simulink model "DC_Motor"  (R2021a)
settings: Solver=FixedStepAuto  StartTime=0.0  StopTime=10.0  FixedStep=25e-6  RelTol=1e-3
undefined symbols (not defined in the file): B, kephi, kphi, Ra, tau_a, tau_m, TL, Va
libraries: simulink_extras x2, spspowerguiLib x1
settings Model: Creator=lesinko morris  LastModifiedBy=lesinko morris
settings DataIOCC: SaveOutput=off  SignalLogging=off  SaveTime=off  ReturnWorkspaceOutputs=off  LoggingToFile=on

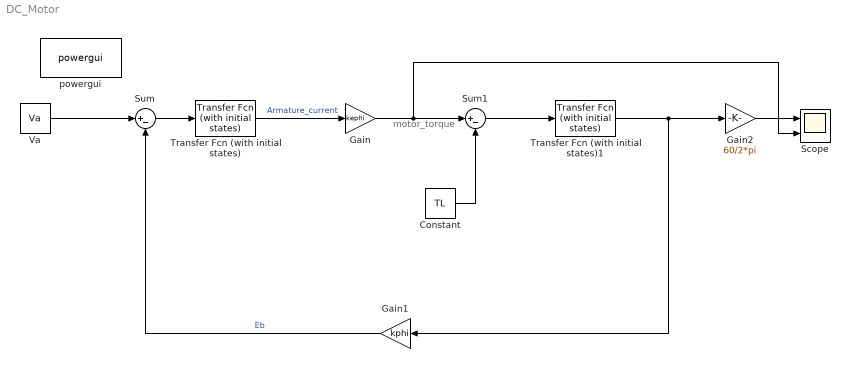
== system DC_Motor ==
  note: motor_torque
  Constant : Constant  Value=TL
  Gain : Gain  Gain=kephi
  Gain1 : Gain  Gain=kphi
  Gain2 : Gain  Gain=60/2*pi
  Scope : Scope  NumInputPorts=2
  Sum : Sum  Inputs=|+-
  Sum1 : Sum  Inputs=|+-
  Transfer Fcn (with initial states) : simulink_extras/Additional Linear/Transfer Fcn (with initial states)  N=[1/Ra]  D=[tau_a 1]  X0=.5
  Transfer Fcn (with initial states)1 : simulink_extras/Additional Linear/Transfer Fcn (with initial states)  N=[1/B]  D=[tau_m 1]  X0=.5
  Va : Constant  Value=Va
  powergui : spspowerguiLib/powergui  Priority=1  SimulationMode=Continuous  SampleTime=50e-6  frequency=60  Iterations=50  frequencyindice=60  Pbase=100e6  ErrMax=1e-4  UnitsV=kV  UnitsW=MW  buscounter=0  FunctionMessages=off  echomessages=off  EnableUseOfTLC=off  CurrentSourceSwitches=off  DisableSnubberDevices=off  DisableRonSwitches=off  DisableVfSwitches=off  DisplayEquations=off  AutomaticDiscreteSolvers=off  SolverType=Tustin/Backward Euler (TBE)  Interpol=off  ExternalGateDelay=off  methode=off  Ts=100  x0status=blocks  SPID=on  SwTol=0  HookPort=off  NonlinearTolerance=1e-4  nMaxIteration=100  ContinueOnMaxIteration=off  RestoreLinks=warning  ResistiveCurrentMeasurement=off  Frange=[0:2:500]  Ylog=off  Xlog=on  ShowGrid=off  save=off  variable=ZData  structure=0  ZoomFFT=off  StartTime=0.0  cycles=1  DisplayStyle=1  fundamental=60  FreqAxis=off  MaxFrequency=1000  frequencyindicesteady=1  RmsSteady=1  display=off
  wires:
  Va/1 -> Sum/1
  Sum/1 -> Transfer Fcn (with initial states)/1
  Transfer Fcn (with initial states)/1 -> Gain/1  "Armature_current"
  Sum1/1 -> Transfer Fcn (with initial states)1/1
  Transfer Fcn (with initial states)1/1 -> Gain1/1, Gain2/1
  Gain1/1 -> Sum/2  "Eb"
  Gain2/1 -> Scope/1
  Gain/1 -> Scope/2, Sum1/1
  Constant/1 -> Sum1/2
